simulink model "integrated_campus_demo"  (Simulink 8.1)
settings: Solver=ode3  SolverMode=SingleTasking  StartTime=0.0  StopTime=24*3600  FixedStep=5  MaxStep=1/60  RelTol=1e-3
PostLoadFcn:
  | % Force reinitialization of Weather block to create bus definition
  | wBlk = [gcs '/Weather Data'];
  | set_param(wBlk,'initbus',get_param(wBlk,'initbus'));
  | clear('wBlk');
undefined symbols (not defined in the file or in its folder): D11, Delta, Ts
libraries: powerlib x41, CampusEnergyModeling x37, powerlib_meascontrol x11, simulink x7
(part 1 of 2)
Description:
  | Copyright 2008-2012 The MathWorks, Inc.
settings Model: Creator=MathWorks  LastModifiedBy=sfrank1  ExtModeTrigMode=oneshot  ExtModeArmWhenConnect=off  ExtModeAutoUpdateStatusClock=off
settings DataIOCC: LimitDataPoints=off  SaveFormat=Structure  SaveOutput=off  SignalLogging=off  DSMLogging=off  SaveTime=off  SignalLoggingName=sigsOut
settings OptimizationCC: BlockReduction=off  BooleanDataType=off  InitFltsAndDblsToZero=on  AccelVerboseBuild=on
settings DebuggingCC: SaveWithParameterizedLinksMsg=none  SignalResolutionControl=TryResolveAllWithWarning  SolverPrmCheckMsg=none  InheritedTsInSrcMsg=none  MultiTaskDSMMsg=warning  MultiTaskCondExecSysMsg=none  UnconnectedLineMsg=none
settings HardwareCC: TargetUnknown=on
settings RTWCC: IncludeERTFirstTime=on
settings GRTTargetCC: TargetFcnLib=ansi_tfl_tmw.mat

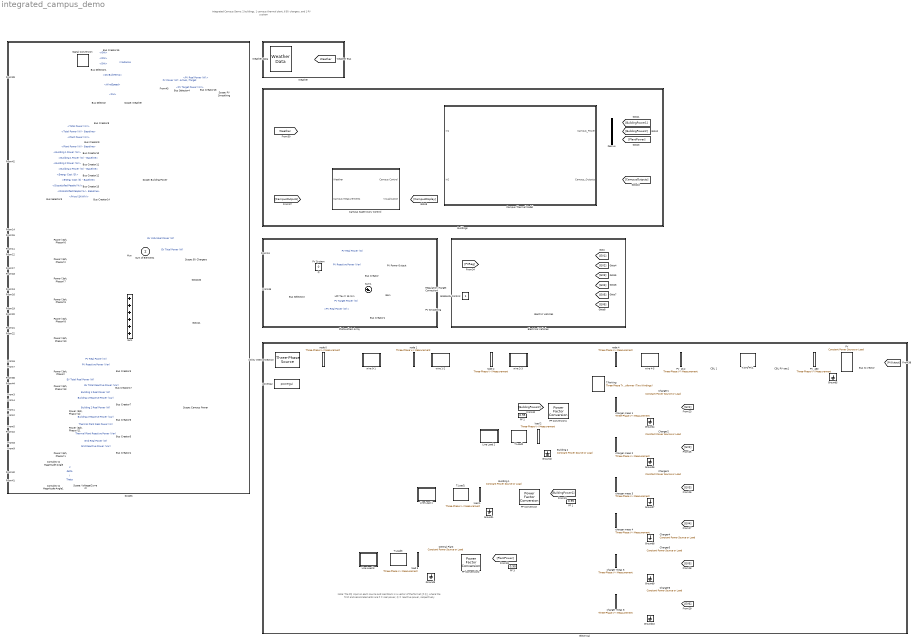
== system integrated_campus_demo ==
  note: Note: The PQ input on each source and load block is a vector of the format [P Q], where the
      | first and second elements are P = real power, Q = reactive power, respectively.
  note: Integrated Campus Demo:
      | 2 buildings, 1 campus thermal plant, 6 EV chargers, and 1 PV system
  Building 1 : CampusEnergyModeling/Electrical/Constant Power Source or Load  Conven=load  PNom=15e3  QNom=5e3  VNom=480  fNom=60  VLow=0.7
  Building 2 : CampusEnergyModeling/Electrical/Constant Power Source or Load  Conven=load  PNom=15e3  QNom=5e3  VNom=480  fNom=60  VLow=0.7
  Buildings : Subsystem
      mask Display: disp('')
  Bus Creator{,1,3..13,16..17} (15 alike) : BusCreator  Inputs=2
  Bus Creator14 : BusCreator  Inputs=1
  Bus Creator15 : BusCreator  Inputs=3
  Bus Selector : BusSelector  OutputSignals=DryBulbTemp,WindSpeed,RH
  Bus Selector1 : BusSelector  OutputSignals=GHI,DNI,DHI
  Bus Selector2 : BusSelector  OutputSignals=PV Real Power (W)
  Bus Selector3 : BusSelector  OutputSignals=Total Power (W),Total Power (W) - Baseline,Plant Power (W),Plant Power (W) - Baseline,Building 1 Power (W),Building 1 Power (W) - Baseline,Building 2 Power (W),Building 2 Power (W) - Baseline,Energy Cost ($),Energy Cost ($) - Baseline,Dissatisfied People (%),Dissatisfied People (%) - Baseline,Price ($/KWh)
  Bus Selector4 : BusSelector  OutputSignals=PV Real Power (W),PV Target Power (W)
  Bus to Vector : BusToVector
  CBL 1 : Subsystem  mask(Short Cable){R1=0.2020, X1=0.0457, R0=0.3211, X0=0.1163, L=50}
      mask prompts: R1 "Positive Sequence R (ohms/1000ft)"; X1 "Positive Sequence XL (ohms/1000ft)"; R0 "Zero Sequence R (ohms/1000ft)"; X0 "Zero Sequence XL (ohms/1000ft)"; L "Line Length (ft)"
      mask help:
      | This block implements a short cable using three phase mutual inductance.
      | Self impedances and mutual impedances are set by entering positive and zero sequences parameters.
      mask Display: plot(0,0,100,100,[20,20,80,80,90,80,80,20,20,10],[50,40,40,50,50,50,61,61,50,50])
  CBL PV-sec1 : Subsystem  mask(Short Cable){R1=0.0276, X1=0.0373, R0=0.0438, X0=0.0999, L=700}
      mask prompts: R1 "Positive Sequence R (ohms/1000ft)"; X1 "Positive Sequence XL (ohms/1000ft)"; R0 "Zero Sequence R (ohms/1000ft)"; X0 "Zero Sequence XL (ohms/1000ft)"; L "Line Length (ft)"
      mask help:
      | This block implements a short cable using three phase mutual inductance.
      | Self impedances and mutual impedances are set by entering positive and zero sequences parameters.
      mask Display: plot(0,0,100,100,[20,20,80,80,90,80,80,20,20,10],[50,40,40,50,50,50,61,61,50,50])
  Campus Supervisory Control : Subsystem
  Campus Thermal Model : Subsystem
      mask Display:
      | image(imread('campus.jpg'));
      | disp('Thermal Campus Model');
      | 
      | % Inputs
      | port_label('input', 1, 'Weather');
      | port_label('input', 2, 'Input');
      | 
      | % Outputs
      | port_label('output', 1, 'Outputs');
      | %port_label('output', 2, 'time');
      | %port_label('output', 3, 'real');
  Central Plant : CampusEnergyModeling/Electrical/Constant Power Source or Load  Conven=load  PNom=12e3  QNom=4e3  VNom=480  fNom=60  VLow=0.7
  Charger{1..6} (6 alike) : CampusEnergyModeling/Electrical/Constant Power Source or Load  Conven=load  PNom=6e3  QNom=2e3  VNom=208  fNom=60  VLow=0.7
  Complex to Magnitude-Angle : ComplexToMagnitudeAngle
  Complex to Magnitude-Angle1 : ComplexToMagnitudeAngle
  Demux : Demux  Outputs=3
  Electric Vehicles : Subsystem
  Electrical : Subsystem
      mask Display: disp('')
  Electrical Vehicles : Subsystem
      mask Display: disp('')
  Enable EV Control : Constant  SampleTime=-1
  Gain : Gain  Gain=-1
  Ground{1..10} (10 alike) : powerlib/Elements/Ground  LConnTagsString=a
  LPF Tau = 15 min : TransferFcn  Denominator=[900 1]
  Line Load 1 : Subsystem  mask(Short Cable){R1=0.1280, X1=0.0507, R0=0.2035, X0=0.1290, L=50}
      mask prompts: R1 "Positive Sequence R (ohms/1000ft)"; X1 "Positive Sequence XL (ohms/1000ft)"; R0 "Zero Sequence R (ohms/1000ft)"; X0 "Zero Sequence XL (ohms/1000ft)"; L "Line Length (ft)"
      mask help:
      | This block implements a short cable using three phase mutual inductance.
      | Self impedances and mutual impedances are set by entering positive and zero sequences parameters.
      mask Display: plot(0,0,100,100,[20,20,80,80,90,80,80,20,20,10],[50,40,40,50,50,50,61,61,50,50])
  Line Load 2 : Subsystem  mask(Short Cable){R1=0.1280, X1=0.0507, R0=0.2035, X0=0.1290, L=50}
      mask prompts: R1 "Positive Sequence R (ohms/1000ft)"; X1 "Positive Sequence XL (ohms/1000ft)"; R0 "Zero Sequence R (ohms/1000ft)"; X0 "Zero Sequence XL (ohms/1000ft)"; L "Line Length (ft)"
      mask help:
      | This block implements a short cable using three phase mutual inductance.
      | Self impedances and mutual impedances are set by entering positive and zero sequences parameters.
      mask Display: plot(0,0,100,100,[20,20,80,80,90,80,80,20,20,10],[50,40,40,50,50,50,61,61,50,50])
  Line Load 3 : Subsystem  mask(Short Cable){R1=0.1280, X1=0.0507, R0=0.2035, X0=0.1290, L=50}
      mask prompts: R1 "Positive Sequence R (ohms/1000ft)"; X1 "Positive Sequence XL (ohms/1000ft)"; R0 "Zero Sequence R (ohms/1000ft)"; X0 "Zero Sequence XL (ohms/1000ft)"; L "Line Length (ft)"
      mask help:
      | This block implements a short cable using three phase mutual inductance.
      | Self impedances and mutual impedances are set by entering positive and zero sequences parameters.
      mask Display: plot(0,0,100,100,[20,20,80,80,90,80,80,20,20,10],[50,40,40,50,50,50,61,61,50,50])
  Mux : Mux  Inputs=6
  PF 1 : Constant  Value=0.95
  PF 2 : Constant  Value=0.95
  PF 3 : Constant  Value=0.90
  PF Conversion : CampusEnergyModeling/Electrical/Power Factor Conversion  pfType=Lagging
  PF Conversion1 : CampusEnergyModeling/Electrical/Power Factor Conversion  pfType=Lagging
  PF Conversion2 : CampusEnergyModeling/Electrical/Power Factor Conversion  pfType=Lagging
  PV : CampusEnergyModeling/Electrical/Constant Power Source or Load  Conven=source  PNom=30e3  QNom=0  VNom=480  fNom=60  VLow=0.7
  PV System : Subsystem
  PV_13.2 : powerlib/Measurements/Three-Phase V-I Measurement  VoltageMeasurement=phase-to-ground  SetLabelV=on  LabelV=Vabc_PV132  Vpu=off  VpuLL=off  CurrentMeasurement=yes  SetLabelI=on  LabelI=Iabc_PV132  Ipu=off  Pbase=1e6  Vbase=25e3  OutputType=Complex  PhasorSimulation=on  PSBequivalent=0
  PV_480 : powerlib/Measurements/Three-Phase V-I Measurement  VoltageMeasurement=phase-to-ground  SetLabelV=on  LabelV=Vabc_PV480  Vpu=off  VpuLL=off  CurrentMeasurement=yes  SetLabelI=on  LabelI=Iabc_PV480  Ipu=off  Pbase=1e6  Vbase=25e3  OutputType=Complex  PhasorSimulation=on  PSBequivalent=0
  Photovoltaic Array : Subsystem
      mask Display: disp('')
  Power (3ph, Phasor){,1..2,6..13} (11 alike) : powerlib_meascontrol/Measurements/Power (3ph, Phasor)
  Q : Constant  Value=0  SampleTime=-1
  "Scope: Building Power " : Scope  NumInputPorts=7
      settings: ShowLegends=on  TimeRange=90000  YMin=0~0~0~0~0~0~0.02  YMax=40000~6000~15000~15000~2~20~0.06  SaveName=ScopeData4
  Scope: Campus Power : Scope  NumInputPorts=6
      settings: ShowLegends=on  TimeRange=90000  YMin=-10000~-10000~-5000~-5000~-5000~-20000  YMax=40000~40000~15000~15000~15000~80000
  Scope: EV Chargers : Scope  NumInputPorts=2
      settings: ShowLegends=on  TimeRange=90000  YMin=-1000~-10000  YMax=7000~40000
  Scope: PV Smoothing : Scope
      settings: ShowLegends=on  TimeRange=90000  YMin=0  YMax=40000  SaveName=ScopeData12
  Scope: Voltage/Current : Scope  NumInputPorts=4
      settings: ShowLegends=on  TimeRange=90000  YMin=390.8~-3~0~-4  YMax=392~2~25~4  SaveName=ScopeData11
  Scope: Weather : Scope  NumInputPorts=4
      settings: ShowLegends=on  TimeRange=90000  YMin=-500~6~0~20  YMax=2000~22~7~70  SaveName=ScopeData7
  Scopes : Subsystem
      mask Display: disp('')
  Signal Conversion : SignalConversion  ConversionOutput=Virtual bus
  Sum : Sum  Inputs=++++++
  Sum of Elements : Sum  Inputs=+
  Sum1 : Sum  Inputs=|+-
  T:Load1 : powerlib/Elements/Three-Phase Transformer (Two Windings)  Winding1Connection=Delta (D11)  UNITS=pu  NominalPower=[50e3 , 60 ]  Winding1=[13.2e3 , 0.01/2 , 0.0566/(120*pi)/2]  Winding2Connection=Yg  Winding2=[480 , 0.01/2 , 0.0566/(120*pi)/2]  SetSaturation=off  Rm=500  Lm=500  Saturation=[ 0,0 ; 0.0024,1.2 ; 1.0,1.52 ]  Hysteresis=off  DataFile='hysteresis'  SetInitialFlux=off  InitialFluxes=[ 0.8 , -0.8 , 0.7 ]  Measurements=None  MoreParameters=off  BreakLoop=off  DataType=off  TransfoNumber=1
  T:Load2 : powerlib/Elements/Three-Phase Transformer (Two Windings)  Winding1Connection=Delta (D11)  UNITS=pu  NominalPower=[50e3 , 60 ]  Winding1=[13.2e3 , 0.01/2 , 0.0566/(120*pi)/2]  Winding2Connection=Yg  Winding2=[480 , 0.01/2 , 0.0566/(120*pi)/2]  SetSaturation=off  Rm=500  Lm=500  Saturation=[ 0,0 ; 0.0024,1.2 ; 1.0,1.52 ]  Hysteresis=off  DataFile='hysteresis'  SetInitialFlux=off  InitialFluxes=[ 0.8 , -0.8 , 0.7 ]  Measurements=None  MoreParameters=off  BreakLoop=off  DataType=off  TransfoNumber=1
  T:Load3 : powerlib/Elements/Three-Phase Transformer (Two Windings)  Winding1Connection=Delta (D11)  UNITS=pu  NominalPower=[50e3 , 60 ]  Winding1=[13.2e3 , 0.01/2 , 0.0566/(120*pi)/2]  Winding2Connection=Yg  Winding2=[480 , 0.01/2 , 0.0566/(120*pi)/2]  SetSaturation=off  Rm=500  Lm=500  Saturation=[ 0,0 ; 0.0024,1.2 ; 1.0,1.52 ]  Hysteresis=off  DataFile='hysteresis'  SetInitialFlux=off  InitialFluxes=[ 0.8 , -0.8 , 0.7 ]  Measurements=None  MoreParameters=off  BreakLoop=off  DataType=off  TransfoNumber=1
  T:Parking : powerlib/Elements/Three-Phase Transformer (Two Windings)  Winding1Connection=Delta (D11)  UNITS=pu  NominalPower=[50e3 , 60 ]  Winding1=[13.2e3 , 0.0242/2 , 0.021/(120*pi)/2]  Winding2Connection=Yg  Winding2=[208 , 0.0242/2 , 0.021/(120*pi)/2]  SetSaturation=off  Rm=500  Lm=500  Saturation=[ 0,0 ; 0.0024,1.2 ; 1.0,1.52 ]  Hysteresis=off  DataFile='hysteresis'  SetInitialFlux=off  InitialFluxes=[ 0.8 , -0.8 , 0.7 ]  Measurements=None  MoreParameters=off  BreakLoop=off  DataType=off  TransfoNumber=1
  T:XF2-PV1 : powerlib/Elements/Three-Phase Transformer (Two Windings)  Winding1Connection=Delta (D11)  UNITS=pu  NominalPower=[50e3 , 60 ]  Winding1=[13.2e3 , 0.01/2 , 0.0566/(120*pi)/2]  Winding2Connection=Yg  Winding2=[480 , 0.01/2 , 0.0566/(120*pi)/2]  SetSaturation=off  Rm=500  Lm=500  Saturation=[ 0,0 ; 0.0024,1.2 ; 1.0,1.52 ]  Hysteresis=off  DataFile='hysteresis'  SetInitialFlux=off  InitialFluxes=[ 0.8 , -0.8 , 0.7 ]  Measurements=None  MoreParameters=off  BreakLoop=off  DataType=off  TransfoNumber=1
  Utility Interconnection : powerlib/Electrical Sources/Three-Phase Source  Voltage=13.2e3  PhaseAngle=0  Frequency=60  InternalConnection=Yg  SpecifyImpedance=on  Resistance=0.8929  Inductance=16.58e-3  ShortCircuitLevel=100e6  BaseVoltage=13.2e3  XRratio=8  BusType=swing  Pref=0  Qref=0  Qmin=-inf  Qmax=inf
  Weather : Subsystem
      mask Display: disp('')
  Weather Data : CampusEnergyModeling/Weather/Weather Data  fname=Weather.mat  initbus=on
  charger meas 1 : powerlib/Measurements/Three-Phase V-I Measurement  VoltageMeasurement=phase-to-ground  SetLabelV=on  LabelV=Vabc_Charger1  Vpu=off  VpuLL=off  CurrentMeasurement=yes  SetLabelI=on  LabelI=Iabc_Charger1  Ipu=off  Pbase=1e6  Vbase=25e3  OutputType=Complex  PhasorSimulation=on  PSBequivalent=0
  charger meas 2 : powerlib/Measurements/Three-Phase V-I Measurement  VoltageMeasurement=phase-to-ground  SetLabelV=on  LabelV=Vabc_Charger2  Vpu=off  VpuLL=off  CurrentMeasurement=yes  SetLabelI=on  LabelI=Iabc_Charger2  Ipu=off  Pbase=1e6  Vbase=25e3  OutputType=Complex  PhasorSimulation=on  PSBequivalent=0
  charger meas 3 : powerlib/Measurements/Three-Phase V-I Measurement  VoltageMeasurement=phase-to-ground  SetLabelV=on  LabelV=Vabc_Charger3  Vpu=off  VpuLL=off  CurrentMeasurement=yes  SetLabelI=on  LabelI=Iabc_Charger3  Ipu=off  Pbase=1e6  Vbase=25e3  OutputType=Complex  PhasorSimulation=on  PSBequivalent=0
  charger meas 4 : powerlib/Measurements/Three-Phase V-I Measurement  VoltageMeasurement=phase-to-ground  SetLabelV=on  LabelV=Vabc_Charger4  Vpu=off  VpuLL=off  CurrentMeasurement=yes  SetLabelI=on  LabelI=Iabc_Charger4  Ipu=off  Pbase=1e6  Vbase=25e3  OutputType=Complex  PhasorSimulation=on  PSBequivalent=0
  charger meas 5 : powerlib/Measurements/Three-Phase V-I Measurement  VoltageMeasurement=phase-to-ground  SetLabelV=on  LabelV=Vabc_Charger5  Vpu=off  VpuLL=off  CurrentMeasurement=yes  SetLabelI=on  LabelI=Iabc_Charger5  Ipu=off  Pbase=1e6  Vbase=25e3  OutputType=Complex  PhasorSimulation=on  PSBequivalent=0
  charger meas 6 : powerlib/Measurements/Three-Phase V-I Measurement  VoltageMeasurement=phase-to-ground  SetLabelV=on  LabelV=Vabc_Charger6  Vpu=off  VpuLL=off  CurrentMeasurement=yes  SetLabelI=on  LabelI=Iabc_Charger6  Ipu=off  Pbase=1e6  Vbase=25e3  OutputType=Complex  PhasorSimulation=on  PSBequivalent=0
  load 1 : powerlib/Measurements/Three-Phase V-I Measurement  VoltageMeasurement=phase-to-ground  SetLabelV=on  LabelV=Vabc_Load1  Vpu=off  VpuLL=off  CurrentMeasurement=yes  SetLabelI=on  LabelI=Iabc_Load1  Ipu=off  Pbase=1e6  Vbase=25e3  OutputType=Complex  PhasorSimulation=on  PSBequivalent=0
  load 2 : powerlib/Measurements/Three-Phase V-I Measurement  VoltageMeasurement=phase-to-ground  SetLabelV=on  LabelV=Vabc_Load2  Vpu=off  VpuLL=off  CurrentMeasurement=yes  SetLabelI=on  LabelI=Iabc_Load2  Ipu=off  Pbase=1e6  Vbase=25e3  OutputType=Complex  PhasorSimulation=on  PSBequivalent=0
  load 3 : powerlib/Measurements/Three-Phase V-I Measurement  VoltageMeasurement=phase-to-ground  SetLabelV=on  LabelV=Vabc_Load3  Vpu=off  VpuLL=off  CurrentMeasurement=yes  SetLabelI=on  LabelI=Iabc_Load3  Ipu=off  Pbase=1e6  Vbase=25e3  OutputType=Complex  PhasorSimulation=on  PSBequivalent=0
  node 0 : powerlib/Measurements/Three-Phase V-I Measurement  VoltageMeasurement=phase-to-ground  SetLabelV=on  LabelV=Vabc_0  Vpu=off  VpuLL=off  CurrentMeasurement=yes  SetLabelI=on  LabelI=Iabc_0  Ipu=off  Pbase=1e6  Vbase=25e3  OutputType=Complex  PhasorSimulation=on  PSBequivalent=0
  node 1 : powerlib/Measurements/Three-Phase V-I Measurement  VoltageMeasurement=phase-to-ground  SetLabelV=on  LabelV=Vabc_1  Vpu=off  VpuLL=off  CurrentMeasurement=yes  SetLabelI=on  LabelI=Iabc_1  Ipu=off  Pbase=1e6  Vbase=25e3  OutputType=Complex  PhasorSimulation=on  PSBequivalent=0
  node 2 : powerlib/Measurements/Three-Phase V-I Measurement  VoltageMeasurement=phase-to-ground  SetLabelV=on  LabelV=Vabc_2  Vpu=off  VpuLL=off  CurrentMeasurement=yes  SetLabelI=on  LabelI=Iabc_2  Ipu=off  Pbase=1e6  Vbase=25e3  OutputType=Complex  PhasorSimulation=on  PSBequivalent=0
  node 4 : powerlib/Measurements/Three-Phase V-I Measurement  VoltageMeasurement=phase-to-ground  SetLabelV=on  LabelV=Vabc_4  Vpu=off  VpuLL=off  CurrentMeasurement=yes  SetLabelI=on  LabelI=Iabc_4  Ipu=off  Pbase=1e6  Vbase=25e3  OutputType=Complex  PhasorSimulation=on  PSBequivalent=0
  powergui : powerlib/powergui  Priority=2  SimulationMode=Phasor  SolverType=Tustin  SampleTime=Ts  frequency=60  SPID=off  DisableSnubberDevices=off  DisableRonSwitches=off  DisableVfSwitches=off  SwTol=0  Interpol=off  DisplayEquations=off  frequencyindice=60  Pbase=100e6  ErrMax=1e-4  Iterations=50  UnitsV=kV  UnitsW=kW  FunctionMessages=off  echomessages=off  HookPort=off  EnableUseOfTLC=off  x0status=blocks  RestoreLinks=warning  ResistiveCurrentMeasurement=off  Frange=[0:2:500]  Ylog=off  Xlog=on  ShowGrid=off  save=off  variable=ZData  structure=Sig1  ZoomFFT=on  StartTime=0.26  cycles=2  DisplayStyle=1  fundamental=60  FreqAxis=off  MaxFrequency=5000  frequencyindicesteady=1  RmsSteady=1  display=off  Ts=0  methode=off
  wire 0-1 : Subsystem  mask(Short Cable){R1=0.0284, X1=0.0421, R0=0.0451, X0=0.1128, L=500}
      mask prompts: R1 "Positive Sequence R (ohms/1000ft)"; X1 "Positive Sequence XL (ohms/1000ft)"; R0 "Zero Sequence R (ohms/1000ft)"; X0 "Zero Sequence XL (ohms/1000ft)"; L "Line Length (ft)"
      mask help:
      | This block implements a short cable using three phase mutual inductance.
      | Self impedances and mutual impedances are set by entering positive and zero sequences parameters.
      mask Display: plot(0,0,100,100,[20,20,80,80,90,80,80,20,20,10],[50,40,40,50,50,50,61,61,50,50])
  wire 1-2 : Subsystem  mask(Short Cable){R1=0.0284, X1=0.0421, R0=0.0451, X0=0.1128, L=500}
      mask prompts: R1 "Positive Sequence R (ohms/1000ft)"; X1 "Positive Sequence XL (ohms/1000ft)"; R0 "Zero Sequence R (ohms/1000ft)"; X0 "Zero Sequence XL (ohms/1000ft)"; L "Line Length (ft)"
      mask help:
      | This block implements a short cable using three phase mutual inductance.
      | Self impedances and mutual impedances are set by entering positive and zero sequences parameters.
      mask Display: plot(0,0,100,100,[20,20,80,80,90,80,80,20,20,10],[50,40,40,50,50,50,61,61,50,50])
  wire 2-3 : Subsystem  mask(Short Cable){R1=0.0284, X1=0.0421, R0=0.0451, X0=0.1128, L=500}
      mask prompts: R1 "Positive Sequence R (ohms/1000ft)"; X1 "Positive Sequence XL (ohms/1000ft)"; R0 "Zero Sequence R (ohms/1000ft)"; X0 "Zero Sequence XL (ohms/1000ft)"; L "Line Length (ft)"
      mask help:
      | This block implements a short cable using three phase mutual inductance.
      | Self impedances and mutual impedances are set by entering positive and zero sequences parameters.
      mask Display: plot(0,0,100,100,[20,20,80,80,90,80,80,20,20,10],[50,40,40,50,50,50,61,61,50,50])
  wire 4-5 : Subsystem  mask(Short Cable){R1=0.0284, X1=0.0421, R0=0.0451, X0=0.1128, L=500}
      mask prompts: R1 "Positive Sequence R (ohms/1000ft)"; X1 "Positive Sequence XL (ohms/1000ft)"; R0 "Zero Sequence R (ohms/1000ft)"; X0 "Zero Sequence XL (ohms/1000ft)"; L "Line Length (ft)"
      mask help:
      | This block implements a short cable using three phase mutual inductance.
      | Self impedances and mutual impedances are set by entering positive and zero sequences parameters.
      mask Display: plot(0,0,100,100,[20,20,80,80,90,80,80,20,20,10],[50,40,40,50,50,50,61,61,50,50])
  tag scope: Weather=global
  wires:
  [Vabc_PV480] -> "Power (3ph, Phasor)"/1
  [Iabc_PV480] -> "Power (3ph, Phasor)"/2
  [EV2] -> Charger2/1
  [EV3] -> Charger3/1
  [EV4] -> Charger4/1
  [EV5] -> Charger5/1
  [EV6] -> Charger6/1
  Q/1 -> Bus Creator/2  "PV Reactive Power (Var)"
  "Power (3ph, Phasor)"/2 -> Bus Creator3/2  "PV Reactive Power (Var)"
  "Power (3ph, Phasor)"/1 -> Bus Creator3/1  "PV Real Power (W)"
  "Power (3ph, Phasor)1"/2 -> Bus Creator4/2  "Grid Reactive Power (Var)"
  [Vabc_0] -> "Power (3ph, Phasor)1"/1
  [Iabc_0] -> "Power (3ph, Phasor)1"/2
  [Vabc_Charger2] -> "Power (3ph, Phasor)2"/1
  [Iabc_Charger2] -> "Power (3ph, Phasor)2"/2
  "Power (3ph, Phasor)2"/1 -> Mux/2
  [Vabc_Charger1] -> "Power (3ph, Phasor)6"/1
  [Iabc_Charger1] -> "Power (3ph, Phasor)6"/2
  "Power (3ph, Phasor)6"/1 -> Mux/1
  [Vabc_Charger3] -> "Power (3ph, Phasor)7"/1
  [Iabc_Charger3] -> "Power (3ph, Phasor)7"/2
  "Power (3ph, Phasor)7"/1 -> Mux/3
  [Vabc_Charger5] -> "Power (3ph, Phasor)8"/1
  [Iabc_Charger5] -> "Power (3ph, Phasor)8"/2
  [Vabc_Charger4] -> "Power (3ph, Phasor)9"/1
  [Iabc_Charger4] -> "Power (3ph, Phasor)9"/2
  "Power (3ph, Phasor)9"/1 -> Mux/4
  [Vabc_Charger6] -> "Power (3ph, Phasor)10"/1
  [Iabc_Charger6] -> "Power (3ph, Phasor)10"/2
  "Power (3ph, Phasor)10"/1 -> Mux/6
  Sum of Elements/1 -> [EV_P], Scope: EV Chargers/2  "EV Total Power (W)"
  Weather Data/1 -> [Weather]
  [Weather] -> PV System/1(Weather)
  [EV1] -> Charger1/1
  Electric Vehicles/1(EV1) -> [EV1]
  Electric Vehicles/2(EV2) -> [EV2]
  Electric Vehicles/3(EV3) -> [EV3]
  Electric Vehicles/4(EV4) -> [EV4]
  Electric Vehicles/5(EV5) -> [EV5]
  Electric Vehicles/6(EV6) -> [EV6]
  PV System/1(PV Power) -> Bus Creator/1  "PV Real Power (W)"
  PF Conversion/1 -> Building 1/1
  [BuildingPower2] -> PF Conversion1/1
  PF 2/1 -> PF Conversion1/2
  Mux/1 -> Sum of Elements/1, Scope: EV Chargers/1  "EV Individual Power (W)"
  "Power (3ph, Phasor)6"/2 -> Sum/1
  "Power (3ph, Phasor)2"/2 -> Sum/2
  "Power (3ph, Phasor)10"/2 -> Sum/6
  "Power (3ph, Phasor)8"/2 -> Sum/5
  "Power (3ph, Phasor)9"/2 -> Sum/4
  "Power (3ph, Phasor)7"/2 -> Sum/3
  "Power (3ph, Phasor)8"/1 -> Mux/5
  Enable EV Control/1 -> Electric Vehicles/2(Enable)
  Bus Selector/1 -> Scope: Weather/2  "<DryBulbTemp>"
  Bus Selector/2 -> Scope: Weather/3  "<WindSpeed>"
  Bus Selector/3 -> Scope: Weather/4  "<RH>"
  "Power (3ph, Phasor)1"/1 -> Bus Creator4/1  "Grid Real Power (W)"
  [PVOutput] -> Bus Selector2/1
  LPF Tau = 15 min/1 -> Bus Creator1/2, Sum1/1  "PV Target Power (W)"
  Sum1/1 -> Gain/1
  [PVReg] -> Electric Vehicles/1(Reg)
  Gain/1 -> [PVReg]
  Sum/1 -> [EV_Q]
  Campus Thermal Model/1(Campus_Power) -> Demux/1
  Demux/1 -> [BuildingPower1]
  Demux/2 -> [BuildingPower2]
  Demux/3 -> [PlantPower]
  [Weather] -> Campus Supervisory Control/1(Weather), Campus Thermal Model/1(In1)
  Campus Supervisory Control/1(Campus Control) -> Campus Thermal Model/2(In2)
  Campus Thermal Model/2(Campus_Outputs) -> [CampusOutputs]
  [Vabc_Load3] -> Complex to Magnitude-Angle/1
  Complex to Magnitude-Angle/1 -> Scope: Voltage/Current/1  "V"
  Complex to Magnitude-Angle/2 -> Scope: Voltage/Current/2  "delta"
  [Iabc_Load3] -> Complex to Magnitude-Angle1/1
  Complex to Magnitude-Angle1/1 -> Scope: Voltage/Current/3  "I"
  Complex to Magnitude-Angle1/2 -> Scope: Voltage/Current/4  "Theta"
  [CampusOutputs] -> Campus Supervisory Control/2(Campus Measurements)
  Campus Supervisory Control/2(Visualization) -> [CampusDisplay]
  Bus Creator15/1 -> Scope: Weather/1  "Irradiance"
  Bus Selector2/1 -> LPF Tau = 15 min/1, Sum1/2, Bus Creator1/1  "<PV Real Power (W)>"
  Bus Creator/1 -> [PVOutput]
  [PVOutput] -> Bus to Vector/1
  Bus to Vector/1 -> PV/1
  Bus Creator1/1 -> [PVSmooth]
  [Weather] -> Signal Conversion/1, Bus Selector/1
  Signal Conversion/1 -> Bus Selector1/1
  Bus Creator3/1 -> Scope: Campus Power/1
  Bus Creator4/1 -> Scope: Campus Power/6
  "Power (3ph, Phasor)11"/2 -> Bus Creator5/2  "Thermal Plant Reactive Power (Var)"
  [Vabc_Load3] -> "Power (3ph, Phasor)11"/1
  [Iabc_Load3] -> "Power (3ph, Phasor)11"/2
  "Power (3ph, Phasor)11"/1 -> Bus Creator5/1  "Thermal Plant Real Power (W)"
  "Power (3ph, Phasor)12"/2 -> Bus Creator6/2  "Building 2 Reactive Power (Var)"
  [Vabc_Load2] -> "Power (3ph, Phasor)12"/1
  [Iabc_Load2] -> "Power (3ph, Phasor)12"/2
  "Power (3ph, Phasor)12"/1 -> Bus Creator6/1  "Building 2 Real Power (W)"
  "Power (3ph, Phasor)13"/2 -> Bus Creator7/2  "Building 1 Reactive Power (Var)"
  [Vabc_Load1] -> "Power (3ph, Phasor)13"/1
  [Iabc_Load1] -> "Power (3ph, Phasor)13"/2
  "Power (3ph, Phasor)13"/1 -> Bus Creator7/1  "Building 1 Real Power (W)"
  Bus Creator7/1 -> Scope: Campus Power/3
  Bus Creator6/1 -> Scope: Campus Power/4
  Bus Creator5/1 -> Scope: Campus Power/5
  Bus Creator16/1 -> Scope: PV Smoothing/1
  [CampusDisplay] -> Bus Selector3/1
  Bus Selector3/1 -> Bus Creator8/1  "<Total Power (W)>"
  Bus Selector3/2 -> Bus Creator8/2  "<Total Power (W) - Baseline>"
  Bus Selector3/3 -> Bus Creator9/1  "<Plant Power (W)>"
  Bus Selector3/4 -> Bus Creator9/2  "<Plant Power (W) - Baseline>"
  Bus Selector3/5 -> Bus Creator10/1  "<Building 1 Power (W)>"
  Bus Selector3/6 -> Bus Creator10/2  "<Building 1 Power (W) - Baseline>"
  Bus Selector3/7 -> Bus Creator11/1  "<Building 2 Power (W)>"
  Bus Selector3/8 -> Bus Creator11/2  "<Building 2 Power (W) - Baseline>"
  Bus Selector3/9 -> Bus Creator12/1  "<Energy Cost ($)>"
  Bus Selector3/10 -> Bus Creator12/2  "<Energy Cost ($) - Baseline>"
  Bus Selector3/11 -> Bus Creator13/1  "<Dissatisfied People (%)>"
  Bus Selector3/12 -> Bus Creator13/2  "<Dissatisfied People (%) - Baseline>"
  Bus Selector3/13 -> Bus Creator14/1  "<Price ($/KWh)>"
  Bus Creator11/1 -> "Scope: Building Power "/4
  Bus Creator8/1 -> "Scope: Building Power "/1
  Bus Creator9/1 -> "Scope: Building Power "/2
  Bus Creator10/1 -> "Scope: Building Power "/3
  Bus Creator12/1 -> "Scope: Building Power "/5
  Bus Creator13/1 -> "Scope: Building Power "/6
  Bus Creator14/1 -> "Scope: Building Power "/7
  Bus Selector1/2 -> Bus Creator15/2  "<DNI>"
  Bus Selector1/1 -> Bus Creator15/1  "<GHI>"
  Bus Selector1/3 -> Bus Creator15/3  "<DHI>"
  [PVSmooth] -> Bus Selector4/1  "PV Power (W): Actual / Target"
  Bus Selector4/1 -> Bus Creator16/1  "<PV Real Power (W)>"
  Bus Selector4/2 -> Bus Creator16/2  "<PV Target Power (W)>"
  [EV_P] -> Bus Creator17/1  "EV Total Real Power (W)"
  [EV_Q] -> Bus Creator17/2  "EV Total Reactive Power (Var)"
  Bus Creator17/1 -> Scope: Campus Power/2
  PF Conversion1/1 -> Building 2/1
  PF 1/1 -> PF Conversion/2
  [BuildingPower1] -> PF Conversion/1
  PF Conversion2/1 -> Central Plant/1
  PF 3/1 -> PF Conversion2/2
  [PlantPower] -> PF Conversion2/1
  connections:
  node 1/LConn2 -- Line Load 1/LConn2 -- wire 0-1/RConn2
  wire 0-1/RConn1 -- Line Load 1/LConn1 -- node 1/LConn1
  node 1/LConn3 -- Line Load 1/LConn3 -- wire 0-1/RConn3
  wire 1-2/LConn1 -- node 1/RConn1
  wire 1-2/LConn2 -- node 1/RConn2
  wire 1-2/LConn3 -- node 1/RConn3
  Building 1/RConn4 -- Ground1/LConn1
  Building 1/RConn2 -- load 1/RConn2
  Building 1/RConn1 -- load 1/RConn1
  Building 1/RConn3 -- load 1/RConn3
  wire 2-3/LConn1 -- node 2/RConn1
  wire 2-3/LConn3 -- node 2/RConn3
  wire 2-3/LConn2 -- node 2/RConn2
  wire 1-2/RConn2 -- node 2/LConn2 -- Line Load 2/LConn2
  wire 1-2/RConn3 -- node 2/LConn3 -- Line Load 2/LConn3
  wire 1-2/RConn1 -- node 2/LConn1 -- Line Load 2/LConn1
  wire 4-5/LConn2 -- node 4/RConn2
  wire 4-5/LConn1 -- node 4/RConn1
  Charger1/RConn3 -- charger meas 1/RConn3
  Charger1/RConn2 -- charger meas 1/RConn2
  Charger1/RConn1 -- charger meas 1/RConn1
  Charger1/RConn4 -- Ground4/LConn1
  wire 4-5/LConn3 -- node 4/RConn3
  PV/RConn4 -- Ground5/LConn1
  wire 2-3/RConn2 -- node 4/LConn2 -- T:Parking/LConn2
  Charger2/RConn4 -- Ground6/LConn1
  Charger3/RConn4 -- Ground7/LConn1
  wire 2-3/RConn1 -- node 4/LConn1 -- T:Parking/LConn1
  wire 2-3/RConn3 -- node 4/LConn3 -- T:Parking/LConn3
  Charger5/RConn4 -- Ground9/LConn1
  Charger6/RConn4 -- Ground10/LConn1
  Charger4/RConn4 -- Ground8/LConn1
  Charger6/RConn2 -- charger meas 6/RConn2
  Charger6/RConn1 -- charger meas 6/RConn1
  Charger6/RConn3 -- charger meas 6/RConn3
  charger meas 5/RConn2 -- Charger5/RConn2
  Charger5/RConn3 -- charger meas 5/RConn3
  Charger4/RConn2 -- charger meas 4/RConn2
  Charger4/RConn1 -- charger meas 4/RConn1
  Charger4/RConn3 -- charger meas 4/RConn3
  Charger3/RConn2 -- charger meas 3/RConn2
  Charger3/RConn3 -- charger meas 3/RConn3
  Charger3/RConn1 -- charger meas 3/RConn1
  Charger2/RConn2 -- charger meas 2/RConn2
  Charger2/RConn1 -- charger meas 2/RConn1
  Charger2/RConn3 -- charger meas 2/RConn3
  T:XF2-PV1/RConn1 -- CBL PV-sec1/LConn1
  T:XF2-PV1/RConn2 -- CBL PV-sec1/LConn2
  T:XF2-PV1/RConn3 -- CBL PV-sec1/LConn3
  CBL PV-sec1/RConn1 -- PV_480/RConn1
  CBL PV-sec1/RConn3 -- PV_480/RConn3
  CBL PV-sec1/RConn2 -- PV_480/RConn2
  T:XF2-PV1/LConn3 -- CBL 1/RConn3
  T:XF2-PV1/LConn2 -- CBL 1/RConn2
  T:XF2-PV1/LConn1 -- CBL 1/RConn1
  PV_13.2/LConn3 -- CBL 1/LConn3
  PV_13.2/LConn1 -- CBL 1/LConn1
  PV_13.2/LConn2 -- CBL 1/LConn2
  PV/RConn1 -- PV_480/LConn1
  PV/RConn3 -- PV_480/LConn3
  PV/RConn2 -- PV_480/LConn2
  wire 4-5/RConn1 -- PV_13.2/RConn1
  wire 4-5/RConn2 -- PV_13.2/RConn2
  wire 4-5/RConn3 -- PV_13.2/RConn3
  T:Load1/LConn2 -- Line Load 1/RConn2
  T:Load1/LConn1 -- Line Load 1/RConn1
  T:Load1/LConn3 -- Line Load 1/RConn3
  T:Load1/RConn2 -- load 1/LConn2
  T:Load1/RConn1 -- load 1/LConn1
  T:Load1/RConn3 -- load 1/LConn3
  T:Load2/LConn2 -- Line Load 2/RConn2
  T:Load2/LConn1 -- Line Load 2/RConn1
  T:Load2/LConn3 -- Line Load 2/RConn3
  Utility Interconnection/RConn2 -- node 0/LConn2
  Utility Interconnection/RConn1 -- node 0/LConn1
  Utility Interconnection/RConn3 -- node 0/LConn3
  node 0/RConn3 -- Line Load 3/LConn3 -- wire 0-1/LConn3
  node 0/RConn2 -- Line Load 3/LConn2 -- wire 0-1/LConn2
  node 0/RConn1 -- Line Load 3/LConn1 -- wire 0-1/LConn1
  T:Load2/RConn1 -- load 2/LConn1
  T:Load2/RConn3 -- load 2/LConn3
  T:Load2/RConn2 -- load 2/LConn2
  Building 2/RConn3 -- load 2/RConn3
  Building 2/RConn1 -- load 2/RConn1
  Building 2/RConn2 -- load 2/RConn2
  Building 2/RConn4 -- Ground2/LConn1
  Central Plant/RConn4 -- Ground3/LConn1
  Central Plant/RConn2 -- load 3/RConn2
  Central Plant/RConn1 -- load 3/RConn1
  Central Plant/RConn3 -- load 3/RConn3
  T:Load3/LConn2 -- Line Load 3/RConn2
  T:Load3/LConn1 -- Line Load 3/RConn1
  T:Load3/LConn3 -- Line Load 3/RConn3
  T:Load3/RConn2 -- load 3/LConn2
  T:Load3/RConn1 -- load 3/LConn1
  T:Load3/RConn3 -- load 3/LConn3
  T:Parking/RConn1 -- charger meas 6/LConn1 -- charger meas 5/LConn1 -- charger meas 4/LConn1 -- charger meas 3/LConn1 -- charger meas 2/LConn1 -- charger meas 1/LConn1
  T:Parking/RConn2 -- charger meas 6/LConn2 -- charger meas 5/LConn2 -- charger meas 4/LConn2 -- charger meas 3/LConn2 -- charger meas 2/LConn2 -- charger meas 1/LConn2
  T:Parking/RConn3 -- charger meas 6/LConn3 -- charger meas 5/LConn3 -- charger meas 4/LConn3 -- charger meas 3/LConn3 -- charger meas 2/LConn3 -- charger meas 1/LConn3
  Charger5/RConn1 -- charger meas 5/RConn1

== system integrated_campus_demo/Buildings ==

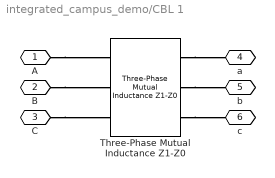
== system integrated_campus_demo/CBL 1 ==
  Three-Phase Mutual Inductance Z1-Z0 : powerlib/Elements/Three-Phase Mutual Inductance Z1-Z0  LConnTagsString=a|b|c  RConnTagsString=A|B|C  PositiveSequence=[R1 X1/376.9911]*L/1000  ZeroSequence=[R0 X0/376.9911]*L/1000
  A : PMIOPort  Port=1  Side=Left
  B : PMIOPort  Port=2  Side=Left
  "C " : PMIOPort  Port=3  Side=Left
  a : PMIOPort  Port=4  Side=Right
  b : PMIOPort  Port=5  Side=Right
  c : PMIOPort  Port=6  Side=Right
  connections:
  Three-Phase Mutual Inductance Z1-Z0/RConn3 -- c/RConn1
  Three-Phase Mutual Inductance Z1-Z0/RConn2 -- b/RConn1
  Three-Phase Mutual Inductance Z1-Z0/RConn1 -- a/RConn1
  "C "/RConn1 -- Three-Phase Mutual Inductance Z1-Z0/LConn3
  B/RConn1 -- Three-Phase Mutual Inductance Z1-Z0/LConn2
  A/RConn1 -- Three-Phase Mutual Inductance Z1-Z0/LConn1

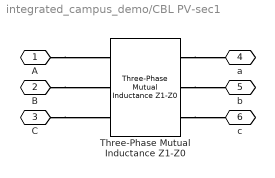
== system integrated_campus_demo/CBL PV-sec1 ==
  Three-Phase Mutual Inductance Z1-Z0 : powerlib/Elements/Three-Phase Mutual Inductance Z1-Z0  LConnTagsString=a|b|c  RConnTagsString=A|B|C  PositiveSequence=[R1 X1/376.9911]*L/1000  ZeroSequence=[R0 X0/376.9911]*L/1000
  A : PMIOPort  Port=1  Side=Left
  B : PMIOPort  Port=2  Side=Left
  "C " : PMIOPort  Port=3  Side=Left
  a : PMIOPort  Port=4  Side=Right
  b : PMIOPort  Port=5  Side=Right
  c : PMIOPort  Port=6  Side=Right
  connections:
  A/RConn1 -- Three-Phase Mutual Inductance Z1-Z0/LConn1
  B/RConn1 -- Three-Phase Mutual Inductance Z1-Z0/LConn2
  "C "/RConn1 -- Three-Phase Mutual Inductance Z1-Z0/LConn3
  Three-Phase Mutual Inductance Z1-Z0/RConn1 -- a/RConn1
  Three-Phase Mutual Inductance Z1-Z0/RConn2 -- b/RConn1
  Three-Phase Mutual Inductance Z1-Z0/RConn3 -- c/RConn1

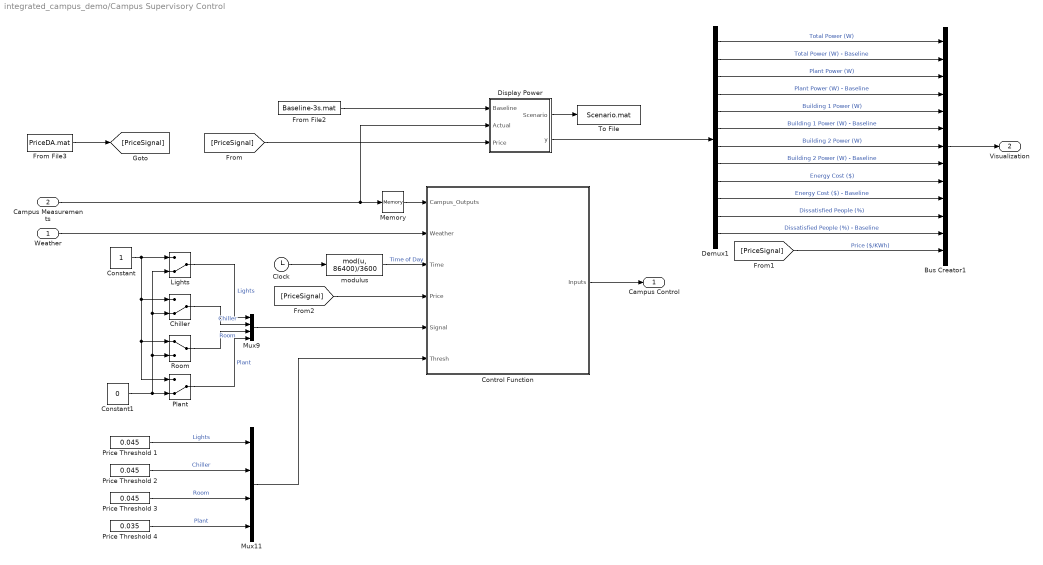
== system integrated_campus_demo/Campus Supervisory Control ==
  Weather : Inport
  Campus Measurements : Inport  Port=2
  Bus Creator1 : BusCreator  Inputs=13
  Chiller : ManualSwitch  CurrentSetting=0
  Clock : Clock
  Constant : Constant
  Constant1 : Constant  Value=0
  Control Function : MATLAB Function  TreatAsAtomicUnit=on
  Demux1 : Demux  Outputs=12
  Display Power : MATLAB Function  TreatAsAtomicUnit=on
  From File2 : FromFile  FileName=Baseline-3s.mat  SampleTime=0
  From File3 : FromFile  FileName=PriceDA.mat  SampleTime=0
  Lights : ManualSwitch  CurrentSetting=0
  Memory : Memory
  Mux11 : Mux
  Mux9 : Mux
  Plant : ManualSwitch  CurrentSetting=0
  Price Threshold 1 : Constant  Value=0.045
  Price Threshold 2 : Constant  Value=0.045
  Price Threshold 3 : Constant  Value=0.045
  Price Threshold 4 : Constant  Value=0.035
  Room : ManualSwitch
  To File : ToFile  Filename=Scenario.mat  SaveFormat=Timeseries
  modulus : MATLABFcn  MATLABFcn=mod(u, 86400)/3600
  Campus Control : Outport
  Visualization : Outport  Port=2
  wires:
  Control Function/1(Inputs) -> Campus Control/1
  Campus Measurements/1 -> Display Power/2(Actual), Memory/1
  Weather/1 -> Control Function/2(Weather)
  Memory/1 -> Control Function/1(Campus_Outputs)
  Clock/1 -> modulus/1
  modulus/1 -> Control Function/3(Time)  "Time of Day"
  Mux9/1 -> Control Function/5(Signal)
  Constant/1 -> Plant/1, Room/1, Chiller/1, Lights/1
  Chiller/1 -> Mux9/2  "Chiller"
  Room/1 -> Mux9/3  "Room"
  Lights/1 -> Mux9/1  "Lights"
  Plant/1 -> Mux9/4  "Plant"
  Constant1/1 -> Lights/2, Chiller/2, Room/2, Plant/2
  Mux11/1 -> Control Function/6(Thresh)
  Price Threshold 1/1 -> Mux11/1  "Lights"
  Price Threshold 2/1 -> Mux11/2  "Chiller"
  Price Threshold 3/1 -> Mux11/3  "Room"
  Price Threshold 4/1 -> Mux11/4  "Plant"
  From File2/1 -> Display Power/1(Baseline)
  [PriceSignal] -> Display Power/3(Price)
  Display Power/2(y) -> Demux1/1
  Display Power/1(Scenario) -> To File/1
  Demux1/1 -> Bus Creator1/1  "Total Power (W)"
  Demux1/2 -> Bus Creator1/2  "Total Power (W) - Baseline"
  Demux1/3 -> Bus Creator1/3  "Plant Power (W)"
  Demux1/4 -> Bus Creator1/4  "Plant Power (W) - Baseline"
  Demux1/5 -> Bus Creator1/5  "Building 1 Power (W)"
  Bus Creator1/1 -> Visualization/1
  [PriceSignal] -> Bus Creator1/13  "Price ($/KWh)"
  From File3/1 -> [PriceSignal]
  [PriceSignal] -> Control Function/4(Price)
  Demux1/6 -> Bus Creator1/6  "Building 1 Power (W) - Baseline"
  Demux1/7 -> Bus Creator1/7  "Building 2 Power (W)"
  Demux1/8 -> Bus Creator1/8  "Building 2 Power (W) - Baseline"
  Demux1/9 -> Bus Creator1/9  "Energy Cost ($)"
  Demux1/10 -> Bus Creator1/10  "Energy Cost ($) - Baseline"
  Demux1/11 -> Bus Creator1/11  "Dissatisfied People (%)"
  Demux1/12 -> Bus Creator1/12  "Dissatisfied People (%) - Baseline"

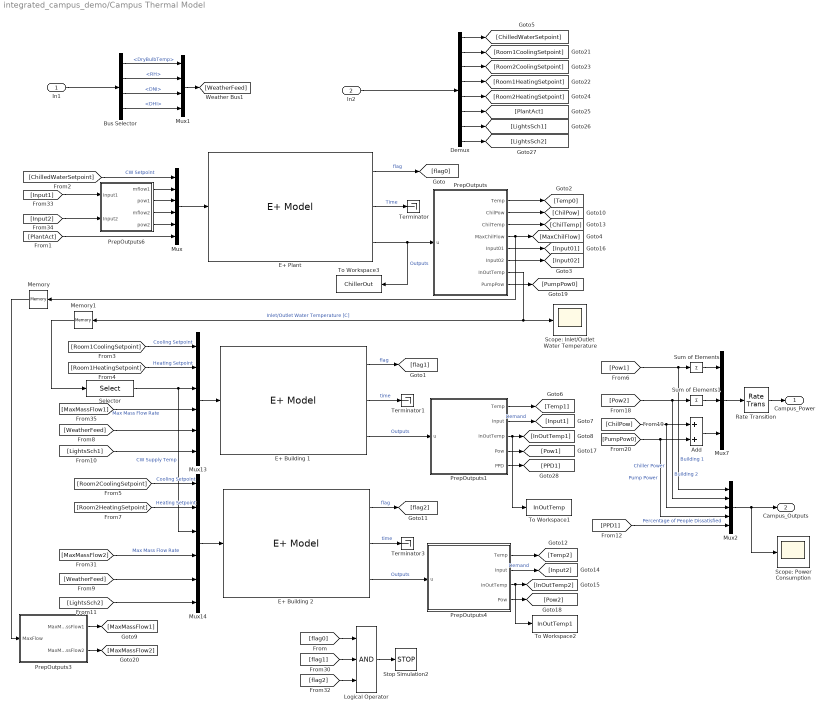
== system integrated_campus_demo/Campus Thermal Model ==
  In1 : Inport
  In2 : Inport  Port=2
  Add : Sum
  Bus Selector : BusSelector  OutputSignals=DryBulbTemp,RH,DNI,DHI
  Demux : Demux  Outputs=8
  E+ Building 1 : CampusEnergyModeling/Buildings/E+ Model  progname='C:\EnergyPlusV8-0-1\RunEPlus.bat'  modelfile=[pwd '\Building1\5ZoneAirCool']  weatherfile='USA_CO_Golden-NREL.724666_TMY3'  workdir=[pwd '\Building1']  timeout=20000  port=0  host=''  bcvtbdir=''  deltaT=60  noutputd=14
  E+ Building 2 : CampusEnergyModeling/Buildings/E+ Model  progname='C:\EnergyPlusV8-0-1\RunEPlus.bat'  modelfile=[pwd '\Building2\5ZoneAirCool']  weatherfile='USA_CO_Golden-NREL.724666_TMY3'  workdir=[pwd '\Building2']  timeout=20000  port=0  host=''  bcvtbdir=''  deltaT=60  noutputd=13
  E+ Plant : CampusEnergyModeling/Buildings/E+ Model  progname='C:\EnergyPlusV8-0-1\RunEPlus.bat'  modelfile=[pwd '\ElectricChiller\ElectricChiller']  weatherfile='USA_CO_Golden-NREL.724666_TMY3'  workdir=[pwd '\ElectricChiller']  timeout=20000  port=0  host=''  bcvtbdir=''  deltaT=60  noutputd=13
  Logical Operator : Logic  Inputs=3  IconShape=distinctive  AllPortsSameDT=off  OutDataTypeStr=boolean
  Memory : Memory
  Memory1 : Memory
  Mux : Mux  Inputs=6
  Mux1 : Mux
  Mux13 : Mux  Inputs=6
  Mux14 : Mux  Inputs=6
  Mux2 : Mux  Inputs=5
  Mux7 : Mux  Inputs=3
  PrepOutputs : MATLAB Function  TreatAsAtomicUnit=on
  PrepOutputs1 : MATLAB Function  TreatAsAtomicUnit=on
  PrepOutputs3 : MATLAB Function  TreatAsAtomicUnit=on
  PrepOutputs4 : MATLAB Function  Priority=2  TreatAsAtomicUnit=on
  PrepOutputs6 : MATLAB Function  TreatAsAtomicUnit=on
  Rate Transition : RateTransition
  Scope: Inlet/Outlet Water Temperature : Scope
      settings: ShowLegends=on  TimeRange=90000  YMin=7  YMax=15  SaveName=ScopeData3
  Scope: Power Consumption : Scope
      settings: ShowLegends=on  TimeRange=90000  YMin=0  YMax=12000  SaveName=ScopeData9
  Selector : Selector  InputPortWidth=4  IndexOptions=Index vector (dialog)  Indices=[1]  OutputSizes=1
  Stop Simulation2 : Stop
  Sum of Elements : Sum  Inputs=+
  Sum of Elements1 : Sum  Inputs=+
  Terminator : Terminator
  Terminator1 : Terminator
  Terminator3 : Terminator
  To Workspace1 : ToWorkspace  VariableName=InOutTemp  SampleTime=-1  SaveFormat=Structure With Time
  To Workspace2 : ToWorkspace  VariableName=InOutTemp1  SampleTime=-1  SaveFormat=Structure With Time
  To Workspace3 : ToWorkspace  VariableName=ChillerOut  SampleTime=-1  SaveFormat=Structure With Time
  Campus_Power : Outport
  Campus_Outputs : Outport  Port=2
  wires:
  E+ Plant/1 -> [flag0]  "flag"
  [ChilledWaterSetpoint] -> Mux/1  "CW Setpoint"
  Mux/1 -> E+ Plant/1
  [Room1CoolingSetpoint] -> Mux13/1  "Cooling Setpoint"
  [Room1HeatingSetpoint] -> Mux13/2  "Heating Setpoint"
  Mux13/1 -> E+ Building 1/1
  E+ Building 1/1 -> [flag1]  "flag"
  Logical Operator/1 -> Stop Simulation2/1
  [flag0] -> Logical Operator/1
  [flag1] -> Logical Operator/2
  E+ Plant/2 -> Terminator/1  "Time"
  E+ Building 1/2 -> Terminator1/1  "time"
  E+ Plant/3 -> To Workspace3/1, PrepOutputs/1(u)  "Outputs"
  E+ Building 1/3 -> PrepOutputs1/1(u)  "Outputs"
  PrepOutputs1/1(Temp) -> [Temp1]
  PrepOutputs1/2(Input) -> [Input1]  "Demand"
  PrepOutputs1/3(InOutTemp) -> To Workspace1/1, [InOutTemp1]
  [MaxMassFlow1] -> Mux13/4  "Max Mass Flow Rate"
  PrepOutputs3/1(MaxMassFlow1) -> [MaxMassFlow1]
  [Room2CoolingSetpoint] -> Mux14/1  "Cooling Setpoint"
  [Room2HeatingSetpoint] -> Mux14/2  "Heating Setpoint"
  Mux14/1 -> E+ Building 2/1
  E+ Building 2/1 -> [flag2]  "flag"
  E+ Building 2/2 -> Terminator3/1  "time"
  E+ Building 2/3 -> PrepOutputs4/1(u)  "Outputs"
  PrepOutputs4/1(Temp) -> [Temp2]
  PrepOutputs4/2(Input) -> [Input2]  "Demand"
  PrepOutputs4/3(InOutTemp) -> [InOutTemp2], To Workspace2/1
  [MaxMassFlow2] -> Mux14/4  "Max Mass Flow Rate"
  [flag2] -> Logical Operator/3
  PrepOutputs/1(Temp) -> [Temp0]
  PrepOutputs/2(ChilPow) -> [ChilPow]
  PrepOutputs/3(ChilTemp) -> [ChilTemp]
  PrepOutputs/5(Input01) -> [Input01]
  PrepOutputs/6(Input02) -> [Input02]
  PrepOutputs1/4(Pow) -> [Pow1]
  PrepOutputs4/4(Pow) -> [Pow2]
  PrepOutputs/8(PumpPow) -> [PumpPow0]
  Selector/1 -> Mux14/3, Mux13/3  "CW Supply Temp"
  PrepOutputs3/2(MaxMassFlow2) -> [MaxMassFlow2]
  PrepOutputs/7(InOutTemp) -> Memory1/1, Scope: Inlet/Outlet Water Temperature/1  "Inlet/Outlet Water Temperature [C]"
  PrepOutputs/4(MaxChilFlow) -> Memory/1, [MaxChilFlow]
  PrepOutputs6/1(mflow1) -> Mux/2
  PrepOutputs6/2(pow1) -> Mux/3
  PrepOutputs6/3(mflow2) -> Mux/4
  PrepOutputs6/4(pow2) -> Mux/5
  [Input1] -> PrepOutputs6/1(Input1)
  [Input2] -> PrepOutputs6/2(Input2)
  Memory/1 -> PrepOutputs3/1(MaxFlow)
  Memory1/1 -> Selector/1
  [Pow1] -> Mux2/1, Sum of Elements/1  "Building 1"
  [Pow2] -> Mux2/2, Sum of Elements1/1  "Building 2"
  Mux7/1 -> Rate Transition/1
  [PumpPow0] -> Mux2/4, Add/2  "Pump Power"
  [ChilPow] -> Mux2/3, Add/1  "Chiller Power"
  Add/1 -> Mux7/3
  Rate Transition/1 -> Campus_Power/1
  Sum of Elements/1 -> Mux7/1
  Sum of Elements1/1 -> Mux7/2
  In2/1 -> Demux/1
  Demux/1 -> [ChilledWaterSetpoint]
  Demux/2 -> [Room1CoolingSetpoint]
  Demux/3 -> [Room2CoolingSetpoint]
  Demux/4 -> [Room1HeatingSetpoint]
  Demux/5 -> [Room2HeatingSetpoint]
  Mux1/1 -> [WeatherFeed]
  [WeatherFeed] -> Mux13/5
  [WeatherFeed] -> Mux14/5
  In1/1 -> Bus Selector/1
  Bus Selector/3 -> Mux1/3  "<DNI>"
  Bus Selector/2 -> Mux1/2  "<RH>"
  Bus Selector/4 -> Mux1/4  "<DHI>"
  Bus Selector/1 -> Mux1/1  "<DryBulbTemp>"
  Mux2/1 -> Scope: Power Consumption/1, Campus_Outputs/1
  Demux/6 -> [PlantAct]
  [PlantAct] -> Mux/6
  [LightsSch1] -> Mux13/6
  [LightsSch2] -> Mux14/6
  Demux/7 -> [LightsSch1]
  Demux/8 -> [LightsSch2]
  PrepOutputs1/5(PPD) -> [PPD1]
  [PPD1] -> Mux2/5  "Percentage of People Dissatisfied"

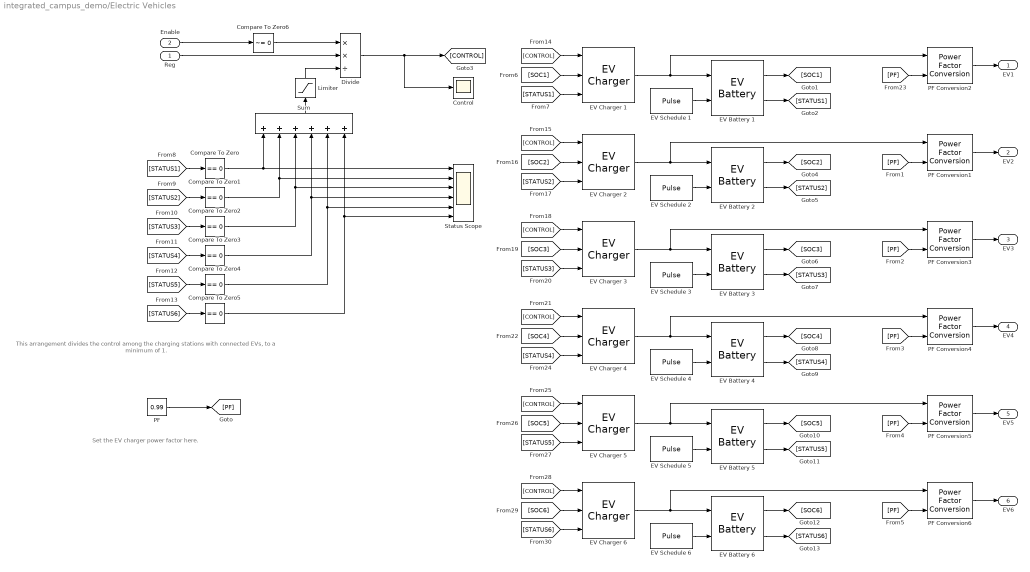
== system integrated_campus_demo/Electric Vehicles ==
  note: This arrangement divides the control among the charging stations with
      | connected EVs, to a minimum of 1.
  note: Set the EV charger power factor here.
  Reg : Inport
  Enable : Inport  Port=2
  Compare To Zero{,1..5} (6 alike) : simulink/Logic and Bit Operations/Compare To Zero  relop===  OutDataTypeStr=boolean
  Compare To Zero6 : simulink/Logic and Bit Operations/Compare To Zero  relop=~=  OutDataTypeStr=boolean
  Control : Scope
      settings: TimeRange=100000  YMin=-12187.5  YMax=12187.5  SaveName=ScopeData5
  Divide : Product  Inputs=**/
  EV Battery {1..6} (6 alike) : CampusEnergyModeling/Electrical/EV Battery  capacity=24000  initSOC=0.3
  EV Charger {1..6} (6 alike) : CampusEnergyModeling/Electrical/EV Charger  rating=6240  capacity=24000  maxresponse=2000  ramp=5000
  EV Schedule {1..6} (6 alike) : DiscretePulseGenerator  Period=24*3600/5  PulseWidth=round((8 + 1*rand(1))*3600/5)  PhaseDelay=round((7 + 2*rand(1))*3600/5)  SampleTime=5
  Limiter : Saturate  UpperLimit=6  LowerLimit=1
  PF : Constant  Value=0.99
  PF Conversion{1..6} (6 alike) : CampusEnergyModeling/Electrical/Power Factor Conversion  pfType=Lagging
  Status Scope : Scope  NumInputPorts=6
      settings: TimeRange=100000  YMin=0~0~0~0~0~0  YMax=1~1~1~1~1~1  SaveName=ScopeData6
  Sum : Sum  Inputs=++++++
  EV1 : Outport
  EV2 : Outport  Port=2
  EV3 : Outport  Port=3
  EV4 : Outport  Port=4
  EV5 : Outport  Port=5
  EV6 : Outport  Port=6
  wires:
  PF Conversion2/1 -> EV1/1
  PF Conversion1/1 -> EV2/1
  PF Conversion3/1 -> EV3/1
  PF Conversion4/1 -> EV4/1
  PF Conversion5/1 -> EV5/1
  PF Conversion6/1 -> EV6/1
  PF/1 -> [PF]
  [PF] -> PF Conversion2/2
  [PF] -> PF Conversion1/2
  [PF] -> PF Conversion3/2
  [PF] -> PF Conversion4/2
  [PF] -> PF Conversion5/2
  [PF] -> PF Conversion6/2
  EV Charger 1/1 -> PF Conversion2/1, EV Battery 1/1
  EV Battery 1/1 -> [SOC1]
  EV Battery 1/2 -> [STATUS1]
  [SOC1] -> EV Charger 1/2
  [STATUS1] -> EV Charger 1/3
  EV Schedule 1/1 -> EV Battery 1/2
  [STATUS1] -> Compare To Zero/1
  Compare To Zero/1 -> Status Scope/1, Sum/1
  [STATUS2] -> Compare To Zero1/1
  [STATUS3] -> Compare To Zero2/1
  [STATUS4] -> Compare To Zero3/1
  [STATUS5] -> Compare To Zero4/1
  [STATUS6] -> Compare To Zero5/1
  Compare To Zero1/1 -> Status Scope/2, Sum/2
  Compare To Zero2/1 -> Status Scope/3, Sum/3
  Compare To Zero3/1 -> Status Scope/4, Sum/4
  Compare To Zero4/1 -> Status Scope/5, Sum/5
  Compare To Zero5/1 -> Status Scope/6, Sum/6
  Sum/1 -> Limiter/1
  Limiter/1 -> Divide/3
  [CONTROL] -> EV Charger 1/1
  EV Charger 2/1 -> PF Conversion1/1, EV Battery 2/1
  EV Battery 2/1 -> [SOC2]
  EV Battery 2/2 -> [STATUS2]
  [SOC2] -> EV Charger 2/2
  [STATUS2] -> EV Charger 2/3
  EV Schedule 2/1 -> EV Battery 2/2
  [CONTROL] -> EV Charger 2/1
  EV Charger 3/1 -> PF Conversion3/1, EV Battery 3/1
  EV Battery 3/1 -> [SOC3]
  EV Battery 3/2 -> [STATUS3]
  [SOC3] -> EV Charger 3/2
  [STATUS3] -> EV Charger 3/3
  EV Schedule 3/1 -> EV Battery 3/2
  [CONTROL] -> EV Charger 3/1
  EV Charger 4/1 -> PF Conversion4/1, EV Battery 4/1
  EV Battery 4/1 -> [SOC4]
  EV Battery 4/2 -> [STATUS4]
  [SOC4] -> EV Charger 4/2
  [STATUS4] -> EV Charger 4/3
  EV Schedule 4/1 -> EV Battery 4/2
  [CONTROL] -> EV Charger 4/1
  EV Charger 5/1 -> PF Conversion5/1, EV Battery 5/1
  EV Battery 5/1 -> [SOC5]
  EV Battery 5/2 -> [STATUS5]
  [SOC5] -> EV Charger 5/2
  [STATUS5] -> EV Charger 5/3
  EV Schedule 5/1 -> EV Battery 5/2
  [CONTROL] -> EV Charger 5/1
  EV Charger 6/1 -> PF Conversion6/1, EV Battery 6/1
  EV Battery 6/1 -> [SOC6]
  EV Battery 6/2 -> [STATUS6]
  [SOC6] -> EV Charger 6/2
  [STATUS6] -> EV Charger 6/3
  EV Schedule 6/1 -> EV Battery 6/2
  [CONTROL] -> EV Charger 6/1
  Reg/1 -> Divide/2
  Enable/1 -> Compare To Zero6/1
  Compare To Zero6/1 -> Divide/1
  Divide/1 -> [CONTROL], Control/1

== system integrated_campus_demo/Electrical ==

== system integrated_campus_demo/Electrical Vehicles ==

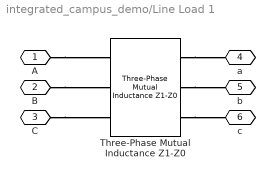
== system integrated_campus_demo/Line Load 1 ==
  Three-Phase Mutual Inductance Z1-Z0 : powerlib/Elements/Three-Phase Mutual Inductance Z1-Z0  LConnTagsString=a|b|c  RConnTagsString=A|B|C  PositiveSequence=[R1 X1/376.9911]*L/1000  ZeroSequence=[R0 X0/376.9911]*L/1000
  A : PMIOPort  Port=1  Side=Left
  B : PMIOPort  Port=2  Side=Left
  "C " : PMIOPort  Port=3  Side=Left
  a : PMIOPort  Port=4  Side=Right
  b : PMIOPort  Port=5  Side=Right
  c : PMIOPort  Port=6  Side=Right
  connections:
  A/RConn1 -- Three-Phase Mutual Inductance Z1-Z0/LConn1
  B/RConn1 -- Three-Phase Mutual Inductance Z1-Z0/LConn2
  "C "/RConn1 -- Three-Phase Mutual Inductance Z1-Z0/LConn3
  Three-Phase Mutual Inductance Z1-Z0/RConn1 -- a/RConn1
  Three-Phase Mutual Inductance Z1-Z0/RConn2 -- b/RConn1
  Three-Phase Mutual Inductance Z1-Z0/RConn3 -- c/RConn1

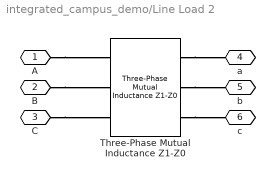
== system integrated_campus_demo/Line Load 2 ==
  Three-Phase Mutual Inductance Z1-Z0 : powerlib/Elements/Three-Phase Mutual Inductance Z1-Z0  LConnTagsString=a|b|c  RConnTagsString=A|B|C  PositiveSequence=[R1 X1/376.9911]*L/1000  ZeroSequence=[R0 X0/376.9911]*L/1000
  A : PMIOPort  Port=1  Side=Left
  B : PMIOPort  Port=2  Side=Left
  "C " : PMIOPort  Port=3  Side=Left
  a : PMIOPort  Port=4  Side=Right
  b : PMIOPort  Port=5  Side=Right
  c : PMIOPort  Port=6  Side=Right
  connections:
  Three-Phase Mutual Inductance Z1-Z0/RConn3 -- c/RConn1
  Three-Phase Mutual Inductance Z1-Z0/RConn2 -- b/RConn1
  Three-Phase Mutual Inductance Z1-Z0/RConn1 -- a/RConn1
  "C "/RConn1 -- Three-Phase Mutual Inductance Z1-Z0/LConn3
  B/RConn1 -- Three-Phase Mutual Inductance Z1-Z0/LConn2
  A/RConn1 -- Three-Phase Mutual Inductance Z1-Z0/LConn1

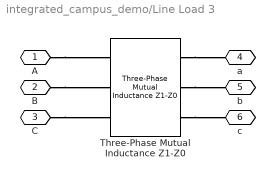
== system integrated_campus_demo/Line Load 3 ==
  Three-Phase Mutual Inductance Z1-Z0 : powerlib/Elements/Three-Phase Mutual Inductance Z1-Z0  LConnTagsString=a|b|c  RConnTagsString=A|B|C  PositiveSequence=[R1 X1/376.9911]*L/1000  ZeroSequence=[R0 X0/376.9911]*L/1000
  A : PMIOPort  Port=1  Side=Left
  B : PMIOPort  Port=2  Side=Left
  "C " : PMIOPort  Port=3  Side=Left
  a : PMIOPort  Port=4  Side=Right
  b : PMIOPort  Port=5  Side=Right
  c : PMIOPort  Port=6  Side=Right
  connections:
  A/RConn1 -- Three-Phase Mutual Inductance Z1-Z0/LConn1
  B/RConn1 -- Three-Phase Mutual Inductance Z1-Z0/LConn2
  "C "/RConn1 -- Three-Phase Mutual Inductance Z1-Z0/LConn3
  Three-Phase Mutual Inductance Z1-Z0/RConn1 -- a/RConn1
  Three-Phase Mutual Inductance Z1-Z0/RConn2 -- b/RConn1
  Three-Phase Mutual Inductance Z1-Z0/RConn3 -- c/RConn1

== system integrated_campus_demo/PV System ==
  Weather : Inport
  Bus Selector : BusSelector  OutputSignals=DNI,DHI,DryBulbTemp,WindSpeed
  PV Powered PVP30KW-480 30 kW inverter : CampusEnergyModeling/PV/Generic Inverter  model_type=Lookup Table  fixed_eff=0.95  alpha=1  beta=0.01  gamma=0.001  lookup_pair=Output Power + Efficiency  lookup_in=[0, 10, 25, 50, 75, 100]  lookup_out=30e3 .* [0, 0.10 0.20, 0.30, 0.50, 0.75, 1.00]  lookup_eff=[50.0, 90.0, 93.6, 94.4, 94.9, 94.6, 94.1] ./ 100
  PVWatts Cosimulation : CampusEnergyModeling/PV/PVWatts Cosimulation  lat=39.74  lon=-105.18  start_time=2012-01-01 00:00:00  tz=-6  time_step=15  system_size=30000  derate=0.95  azimuth=180  tilt=39.74  use_lat_tilt=on  track_mode=Fixed  rotlim=45  use_cell_data=off  t_ref=25  t_noct=45  gamma=-0.5  i_ref=1000  poa_cutin=0  init_tcell=25  init_poa=0  output_dc=on  output_celltemp=off  output_poa=off
  Rate Limiter : RateLimiter  RisingSlewLimit=5e3  FallingSlewLimit=-5e3  SampleTimeMode=inherited
  PV Power : Outport
  wires:
  PV Powered PVP30KW-480 30 kW inverter/1 -> Rate Limiter/1
  PVWatts Cosimulation/1 -> PV Powered PVP30KW-480 30 kW inverter/1
  Weather/1 -> Bus Selector/1
  Bus Selector/1 -> PVWatts Cosimulation/1  "<DNI>"
  Bus Selector/2 -> PVWatts Cosimulation/2  "<DHI>"
  Bus Selector/3 -> PVWatts Cosimulation/3  "<DryBulbTemp>"
  Bus Selector/4 -> PVWatts Cosimulation/4  "<WindSpeed>"
  Rate Limiter/1 -> PV Power/1

== system integrated_campus_demo/Photovoltaic Array ==

== system integrated_campus_demo/Scopes ==

== system integrated_campus_demo/Weather ==

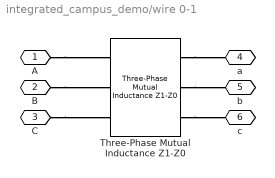
== system integrated_campus_demo/wire 0-1 ==
  Three-Phase Mutual Inductance Z1-Z0 : powerlib/Elements/Three-Phase Mutual Inductance Z1-Z0  LConnTagsString=a|b|c  RConnTagsString=A|B|C  PositiveSequence=[R1 X1/376.9911]*L/1000  ZeroSequence=[R0 X0/376.9911]*L/1000
  A : PMIOPort  Port=1  Side=Left
  B : PMIOPort  Port=2  Side=Left
  "C " : PMIOPort  Port=3  Side=Left
  a : PMIOPort  Port=4  Side=Right
  b : PMIOPort  Port=5  Side=Right
  c : PMIOPort  Port=6  Side=Right
  connections:
  A/RConn1 -- Three-Phase Mutual Inductance Z1-Z0/LConn1
  B/RConn1 -- Three-Phase Mutual Inductance Z1-Z0/LConn2
  "C "/RConn1 -- Three-Phase Mutual Inductance Z1-Z0/LConn3
  Three-Phase Mutual Inductance Z1-Z0/RConn1 -- a/RConn1
  Three-Phase Mutual Inductance Z1-Z0/RConn2 -- b/RConn1
  Three-Phase Mutual Inductance Z1-Z0/RConn3 -- c/RConn1
